simulink library "powerlib_modelsV2"  (Simulink 6.0)
settings: Solver=ode45  SolverMode=SingleTasking  StartTime=0.0  StopTime=10.0  RelTol=1e-3
values from neighbouring files (symbols this model uses):
  Ts = get(handles.edit1,'string')    [powergui.m]
undefined symbols (not defined in the file or in its folder): A, Ac, B, Bc, C, Cc, Cs, Current, damp, Dc, Dd, DiscIntNeverNeededParam, dref, dwo, exc, F, fb, gate, GH, GHd, GI, GId, GL, GLd, H, HT, hyd, ib, ib2, io, isfinite, j, K, Kd, Kg, L, Lad, Laq, lim, LIM, Ll, Llfd, Llkd, Llkq1, Llkq2, Llr, Lls, LowerFlux, N, N2, Nb, Nb2, nb_arm, p, Par_HarmoA_pu, Par_HarmoB_pu, Par_Timing_Harmo, Par_Timing_Variation, Par_Vps, Pb ... (+57)
libraries: powerlib_extras x14
(part 10 of 11)

== system powerlib_modelsV2/Switch Current Source/gto/Conduction Logic ==
  iak : Inport  Port=1  LatchInput=off
  Vak : Inport  Port=2  LatchInput=off
  g : Inport  Port=3  LatchInput=off
  "      " : Constant  Value=0
  ". " : Logic
  . 1 : Logic  Operator=OR
  Break Alg. Loop : Subsystem  mask{Nsw=length(Ron)}
      mask prompts: Nsw "number of switches"
  Data Type  Conversion{1..3,5..6} (5 alike) : DataTypeConversion  SaturateOnIntegerOverflow=on  RndMeth=Zero
  I>0 : Relay  OnSwitchValue=1000*eps  OffSwitchValue=0
  I>1.5 : Relay  OnSwitchValue=1.5  OffSwitchValue=0
  Test2 : Switch  Threshold=eps  InputSameDT=on
  Vf : Constant  Value=Vf
  b : RelationalOperator  Operator=>  InputSameDT=on
  n1 : Sum  SaturateOnIntegerOverflow=on  InputSameDT=on
  status : Outport  InitialOutput=0
  wires:
  Data Type  Conversion5/1 -> Test2/2, ". "/2
  Break Alg. Loop/1(Out1) -> Data Type  Conversion3/1, n1/2
  ". "/1 -> Break Alg. Loop/1(In1)
  Data Type  Conversion3/1 -> . 1/2
  Data Type  Conversion2/1 -> . 1/1
  I>1.5/1 -> Data Type  Conversion2/1
  Data Type  Conversion1/1 -> Test2/1
  . 1/1 -> Data Type  Conversion1/1
  n1/1 -> I>1.5/1
  iak/1 -> I>0/1
  I>0/1 -> n1/1
  Vf/1 -> b/2
  "      "/1 -> Test2/3
  Test2/1 -> status/1
  g/1 -> Data Type  Conversion5/1  "gate signal"
  Data Type  Conversion6/1 -> ". "/1
  b/1 -> Data Type  Conversion6/1
  Vak/1 -> b/1

== system powerlib_modelsV2/Switch Current Source/gto/Tail ==
  iak : Inport  Port=1  LatchInput=off
  switch : Inport  Port=2  LatchInput=off
  1 : Constant
  Integrator : Integrator  ExternalReset=falling  LimitOutput=on
  Look-Up  Table : Lookup  DialogController=Simulink.DDGSource  InputValues="[  0   Tf+eps Tf+Tt+2*eps  Tf+Tt+3*eps]"  OutputValues="[  1   0.1*(Tt>0) 0 0]"  SaturateOnIntegerOverflow=on
  Product : Product  SaturateOnIntegerOverflow=on  InputSameDT=on
  Switch : Switch  Threshold=eps  InputSameDT=on
  Iak : Outport  InitialOutput=0
  wires:
  iak/1 -> Product/1, Switch/1
  Look-Up  Table/1 -> Product/2
  switch/1 -> Switch/2, Integrator/2
  1/1 -> Integrator/1
  Integrator/1 -> Look-Up  Table/1
  Switch/1 -> Iak/1
  Product/1 -> Switch/3

== system powerlib_modelsV2/Switch Current Source/mosfet/Conduction Logic ==
  Ids_meas : Inport  Port=1  LatchInput=off
  Vds : Inport  Port=2  LatchInput=off
  G : Inport  Port=3  LatchInput=off
  "      1" : Constant
  . 1 : Logic  Operator=OR
  . 2 : Logic
  . 3 : Logic  Operator=NOT  Inputs=1
  Break Alg. Loop : Subsystem  mask{Nsw=length(Ron)}
      mask prompts: Nsw "number of switches"
  Data Type  Conversion{,1..2,4..5} (5 alike) : DataTypeConversion  SaturateOnIntegerOverflow=on  RndMeth=Zero
  Test2 : Switch  Threshold=eps  InputSameDT=on
  test_v : RelationalOperator  Operator=<  InputSameDT=on
  test_v1 : RelationalOperator  Operator=<  InputSameDT=on
  zero : Constant  Value=-eps
  zero1 : Constant  Value=-eps
  status : Outport  InitialOutput=0
  wires:
  Break Alg. Loop/1(Out1) -> Data Type  Conversion2/1
  "      1"/1 -> Test2/1
  Test2/1 -> status/1
  Data Type  Conversion/1 -> Test2/3
  test_v/1 -> Data Type  Conversion4/1
  Data Type  Conversion1/1 -> Test2/2, . 3/1
  Data Type  Conversion5/1 -> . 1/1
  test_v1/1 -> Data Type  Conversion5/1
  Data Type  Conversion4/1 -> . 2/1
  zero1/1 -> test_v1/2
  Ids_meas/1 -> test_v1/1
  zero/1 -> test_v/2
  . 2/1 -> Break Alg. Loop/1(In1)
  . 3/1 -> . 2/2
  . 1/1 -> Data Type  Conversion/1
  G/1 -> Data Type  Conversion1/1
  Vds/1 -> test_v/1
  Data Type  Conversion2/1 -> . 1/2

== system powerlib_modelsV2/Switch Current Source/thyristor/Conduction Logic ==
  "Iak " : Inport  Port=1  LatchInput=off
  Vak : Inport  Port=2  LatchInput=off
  "G " : Inport  Port=3  LatchInput=off
  0 1 : Constant  Value=0
  0 2 : Constant  Value=Vf
  0 3 : Constant  Value=0
  Break Alg. Loop : Subsystem  AncestorBlock=powerlib_models/Switch Current Source/thyristor/Conduction Logic/BAL-PB1  mask{Nsw=length(Lon), IC=IC}
      mask prompts: Nsw "number of switches"; IC "initial conditions"
  Data Type  Conversion{1..2,4,6} (4 alike) : DataTypeConversion  SaturateOnIntegerOverflow=on  RndMeth=Zero
  b5 : RelationalOperator  Operator=>  InputSameDT=on
  b6 : RelationalOperator  Operator=>  InputSameDT=on
  b7 : RelationalOperator  Operator===  InputSameDT=on
  or2 : Logic  Operator=OR
  or3 : Logic  Inputs=3
  Status : Outport  InitialOutput=0
  wires:
  Data Type  Conversion4/1 -> or3/3
  or3/1 -> or2/2
  or2/1 -> Break Alg. Loop/1(In1)
  b6/1 -> Data Type  Conversion2/1  "Voltage > Vf"
  b5/1 -> Data Type  Conversion1/1  "Current > 0"
  Vak/1 -> b6/1  "thyristor voltage"
  0 1/1 -> b5/2
  b7/1 -> Data Type  Conversion6/1  "Current = 0"
  0 3/1 -> b7/2
  0 2/1 -> b6/2
  "Iak "/1 -> b7/1, b5/1  "thyristor current"
  "G "/1 -> Data Type  Conversion4/1  "gate signal"
  Data Type  Conversion6/1 -> or3/2
  Data Type  Conversion1/1 -> or2/1
  Data Type  Conversion2/1 -> or3/1
  Break Alg. Loop/1(Out1) -> Status/1

== system powerlib_modelsV2/Continuous/Dynamic_Load/3-phase PLL1/2nd-Order Filter ==
  In : Inport  Port=1  LatchInput=off
  State-Space : StateSpace  A=Ac  B=Bc  C=Cc  D=Dc  X0=x0c
  Out : Outport  InitialOutput=0
  wires:
  State-Space/1 -> Out/1
  In/1 -> State-Space/1

== system powerlib_modelsV2/Continuous/Dynamic_Load/3-phase PLL1/Discrete PI Controller ==
  Error : Inport  Port=1  LatchInput=off
  Integrator : Integrator  InitialCondition=Init  LimitOutput=on  UpperSaturationLimit=UpperLimit  LowerSaturationLimit=LowerLimit
  Kp4 : Gain  Gain=Kp  SaturateOnIntegerOverflow=on
  Kp5 : Gain  Gain=Ki  SaturateOnIntegerOverflow=on
  Saturation2 : Saturate  UpperLimit=UpperLimit  LowerLimit=LowerLimit
  Sum6 : Sum  SaturateOnIntegerOverflow=on  InputSameDT=on
  Out : Outport  InitialOutput=0
  wires:
  Error/1 -> Kp4/1, Kp5/1
  Sum6/1 -> Saturation2/1
  Kp5/1 -> Integrator/1
  Kp4/1 -> Sum6/1
  Integrator/1 -> Sum6/2
  Saturation2/1 -> Out/1

== system powerlib_modelsV2/Continuous/Dynamic_Load/3-phase PLL1/Variable Frequency Mean value ==
  note: Mean Value (Variable frequency)
  note: Pierre Giroux, Gilbert Sybille
      | Power System Simulation Laboratory
      | IREQ, Hydro-Quebc
  Freq : Inport  Port=1  LatchInput=off
  In : Inport  Port=2  LatchInput=off
  Constant : Constant  Value=Vinit
  Integrator : Integrator
  Number of samples per cycle : Fcn  Expr=1/u[1]
  Product : Product  SaturateOnIntegerOverflow=on  InputSameDT=on
  Step : Step  Time=1/Finit  SampleTime=0
  Sum7 : Sum  Inputs=-+  SaturateOnIntegerOverflow=on  InputSameDT=on
  Switch : Switch  Threshold=0.5  InputSameDT=on
  To avoid division by zero : Saturate  Orientation=down  UpperLimit=1e6  LowerLimit=1e-6
  Variable Transport Delay : VariableTransportDelay  MaximumDelay=1/40  MaximumPoints=4096
  Mean : Outport
  wires:
  Number of samples per cycle/1 -> Variable Transport Delay/2  "Delay"
  Step/1 -> Switch/2
  To avoid division by zero/1 -> Number of samples per cycle/1  "Freq"
  Switch/1 -> Mean/1
  Constant/1 -> Switch/3
  Freq/1 -> To avoid division by zero/1, Product/2  "Freq"
  Integrator/1 -> Variable Transport Delay/1, Sum7/2
  Sum7/1 -> Product/1
  Variable Transport Delay/1 -> Sum7/1
  Product/1 -> Switch/1  "Mean value"
  In/1 -> Integrator/1  "In"

== system powerlib_modelsV2/Continuous/Dynamic_Load/3-phase PLL1/abc_to_dq1 ==
  note: This subsystem converts Vab and Vbc to Vd,Vq
  Vab_bc : Inport  Port=1  LatchInput=off
  sin_cos : Inport  Port=2  LatchInput=off
  Fcn2 : Fcn  Expr=(u[4]*(2*u[1]+u[2]) + (sqrt(3)*u[2]*u[3]))/3
  Fcn3 : Fcn  Expr=(u[3]*(2*u[1]+u[2]) + (-sqrt(3)*u[2]*u[4]))/3
  Mux1 : Mux  Inputs=[ 2 2 ]
  vd : Outport  InitialOutput=0
  vq : Outport  Port=2  InitialOutput=0
  wires:
  Vab_bc/1 -> Mux1/1
  Mux1/1 -> Fcn2/1, Fcn3/1
  sin_cos/1 -> Mux1/2
  Fcn2/1 -> vq/1
  Fcn3/1 -> vd/1

== system powerlib_modelsV2/Continuous/Dynamic_Load/Break  Alg. Loop/imag ==
  In1 : Inport  Port=1  LatchInput=off
  State Space : StateSpace  A=A  B=B  C=C  D=Dd  X0=X0
  Out1 : Outport  InitialOutput=0
  wires:
  In1/1 -> State Space/1
  State Space/1 -> Out1/1

== system powerlib_modelsV2/Continuous/Dynamic_Load/Break  Alg. Loop/real ==
  In1 : Inport  Port=1  LatchInput=off
  State Space : StateSpace  A=A  B=B  C=C  D=Dd  X0=X0
  Out1 : Outport  InitialOutput=0
  wires:
  In1/1 -> State Space/1
  State Space/1 -> Out1/1

== system powerlib_modelsV2/Continuous/Dynamic_Load/Positive Sequence  current/TF_P ==
  In1 : Inport  Port=1  LatchInput=off
  State-Space : StateSpace  A=Ac  B=Bc  C=Cc  D=Dc  X0=x0c
  Out1 : Outport
  wires:
  In1/1 -> State-Space/1
  State-Space/1 -> Out1/1

== system powerlib_modelsV2/Continuous/Dynamic_Load/Positive Sequence  current/TF_Q ==
  In1 : Inport  Port=1  LatchInput=off
  State-Space : StateSpace  A=Ac  B=Bc  C=Cc  D=Dc  X0=x0c
  Out1 : Outport
  wires:
  State-Space/1 -> Out1/1
  In1/1 -> State-Space/1

== system powerlib_modelsV2/Continuous/GTO-IGBT Bridge/Diode Logic/Blocking Diodes ==
  G : Inport  Port=1  LatchInput=off
  Bloque D214365 : Selector  Elements=Selec_Diode  InputPortWidth=nb_switch
  Logical Operator : Logic  Operator=NOT
  Memory : Memory  InheritSampleTime=on
  Pulse 1 step : Logic
  Block.D : Outport
  wires:
  Bloque D214365/1 -> Block.D/1
  Pulse 1 step/1 -> Bloque D214365/1  "Blockinkg"
  Memory/1 -> Logical Operator/1
  Logical Operator/1 -> Pulse 1 step/1
  G/1 -> Memory/1, Pulse 1 step/2

== system powerlib_modelsV2/Continuous/GTO-IGBT Bridge/Diode Logic/Trig.  Diodes (No Snubber Capacitance) ==
  G : Inport  Port=1  LatchInput=off
  Ipos : Inport  Port=2  LatchInput=off
  Enable : EnablePort  StatesWhenEnabling=reset
  Data Type  Conversion3 : DataTypeConversion  SaturateOnIntegerOverflow=on  RndMeth=Zero
  Logical Operator : Logic  Operator=NOT
  Memory : Memory  InheritSampleTime=on
  Pulse 1 step : Logic  Inputs=3
  Trig D214365 : Selector  Elements=Selec_Diode  InputPortWidth=nb_switch
  Trig D : Outport
  wires:
  Trig D214365/1 -> Trig D/1
  Pulse 1 step/1 -> Trig D214365/1
  Memory/1 -> Pulse 1 step/2
  Logical Operator/1 -> Pulse 1 step/1
  G/1 -> Memory/1, Logical Operator/1
  Ipos/1 -> Data Type  Conversion3/1
  Data Type  Conversion3/1 -> Pulse 1 step/3

== system powerlib_modelsV2/Continuous/MBPSS/Transfer function for detailed model (HF)/Transfer functions for detailed stabilizer ==
  In1 : Inport  Port=1  LatchInput=off
  Enable : EnablePort
  HF2 : TransferFcn  Numerator=[TH3 1]  Denominator=[TH4 1]
  HF3 : TransferFcn  Numerator=[TH5 1]  Denominator=[TH6 1]
  Out1 : Outport
  wires:
  In1/1 -> HF2/1
  HF3/1 -> Out1/1
  HF2/1 -> HF3/1

== system powerlib_modelsV2/Continuous/MBPSS/Transfer function for detailed model (HF)/Transfer functions for detailed stabilizer2 ==
  In1 : Inport  Port=1  LatchInput=off
  Enable : EnablePort
  HF5 : TransferFcn  Numerator=[TH9 1]  Denominator=[TH10 1]
  HF6 : TransferFcn  Numerator=[TH11 1]  Denominator=[TH12 1]
  Out1 : Outport
  wires:
  HF6/1 -> Out1/1
  In1/1 -> HF5/1
  HF5/1 -> HF6/1

== system powerlib_modelsV2/Continuous/MBPSS/Transfer function for detailed model (IF)/Transfer functions for detailed stabilizer ==
  In1 : Inport  Port=1  LatchInput=off
  Enable : EnablePort
  IF2 : TransferFcn  Numerator=[TI3 1]  Denominator=[TI4 1]
  IF3 : TransferFcn  Numerator=[TI5 1]  Denominator=[TI6 1]
  Out1 : Outport
  wires:
  IF3/1 -> Out1/1
  IF2/1 -> IF3/1
  In1/1 -> IF2/1

== system powerlib_modelsV2/Continuous/MBPSS/Transfer function for detailed model (IF)/Transfer functions for detailed stabilizer2 ==
  In1 : Inport  Port=1  LatchInput=off
  Enable : EnablePort
  IF5 : TransferFcn  Numerator=[TI9 1]  Denominator=[TI10 1]
  IF6 : TransferFcn  Numerator=[TI11 1]  Denominator=[TI12 1]
  Out1 : Outport
  wires:
  In1/1 -> IF5/1
  IF6/1 -> Out1/1
  IF5/1 -> IF6/1

== system powerlib_modelsV2/Continuous/MBPSS/Transfer function for detailed model (LF)/Transfer functions for detailed stabilizer ==
  In1 : Inport  Port=1  LatchInput=off
  Enable : EnablePort
  BF2 : TransferFcn  Numerator=[TL3 1]  Denominator=[TL4 1]
  BF3 : TransferFcn  Numerator=[TL5 1]  Denominator=[TL6 1]
  Out1 : Outport
  wires:
  BF2/1 -> BF3/1
  In1/1 -> BF2/1
  BF3/1 -> Out1/1

== system powerlib_modelsV2/Continuous/MBPSS/Transfer function for detailed model (LF)/Transfer functions for detailed stabilizer2 ==
  In1 : Inport  Port=1  LatchInput=off
  Enable : EnablePort
  BF5 : TransferFcn  Numerator=[TL9 1]  Denominator=[TL10 1]
  BF6 : TransferFcn  Numerator=[TL11 1]  Denominator=[TL12 1]
  Out1 : Outport
  wires:
  BF6/1 -> Out1/1
  In1/1 -> BF5/1
  BF5/1 -> BF6/1

== system powerlib_modelsV2/Continuous/PM_synchronous_machine/iq,id/id ==
  iq : Inport  Port=1  LatchInput=off
  we : Inport  Port=2  LatchInput=off
  vd : Inport  Port=3  LatchInput=off
  1/Ld : Gain  Gain=1/Ld  SaturateOnIntegerOverflow=on
  Lq/Ld : Gain  Gain=Lq/Ld  SaturateOnIntegerOverflow=on
  Product : Product  SaturateOnIntegerOverflow=on  InputSameDT=on
  R/Ld : Gain  Gain=R/Ld  SaturateOnIntegerOverflow=on
  Sum : Sum  Inputs=-++  SaturateOnIntegerOverflow=on  InputSameDT=on
  "id " : Integrator
  id : Outport  InitialOutput=0
  wires:
  1/Ld/1 -> Sum/2
  R/Ld/1 -> Sum/1
  Lq/Ld/1 -> Sum/3
  Sum/1 -> "id "/1
  Product/1 -> Lq/Ld/1
  "id "/1 -> R/Ld/1, id/1
  vd/1 -> 1/Ld/1
  we/1 -> Product/1
  iq/1 -> Product/2

== system powerlib_modelsV2/Continuous/PM_synchronous_machine/iq,id/iq ==
  vq : Inport  Port=1  LatchInput=off
  we : Inport  Port=2  LatchInput=off
  id : Inport  Port=3  LatchInput=off
  1/Lq : Gain  Gain=1/Lq  SaturateOnIntegerOverflow=on
  Ld/Lq : Gain  Gain=Ld/Lq  SaturateOnIntegerOverflow=on
  Product1 : Product  SaturateOnIntegerOverflow=on  InputSameDT=on
  R/Lq : Gain  Gain=R/Lq  SaturateOnIntegerOverflow=on
  Sum1 : Sum  Inputs=---+  SaturateOnIntegerOverflow=on  InputSameDT=on
  "iq " : Integrator
  lam/Lq : Gain  Gain=lam/Lq  SaturateOnIntegerOverflow=on
  iq : Outport  InitialOutput=0
  wires:
  R/Lq/1 -> Sum1/1
  Ld/Lq/1 -> Sum1/2
  lam/Lq/1 -> Sum1/3
  Sum1/1 -> "iq "/1
  Product1/1 -> Ld/Lq/1
  1/Lq/1 -> Sum1/4
  id/1 -> Product1/1
  vq/1 -> 1/Lq/1
  we/1 -> Product1/2, lam/Lq/1
  "iq "/1 -> R/Lq/1, iq/1

== system powerlib_modelsV2/Continuous/Three-Level Bridge/2-level GTO-IGBT Bridge  Logic (modified)/Diode Logic ==
  Vak : Inport  Port=1  LatchInput=off
  G : Inport  Port=2  LatchInput=off
  0 2 : Constant  Value=0
  1 : Logic
  Blocking Diodes : Subsystem
  Data Type  Conversion5 : DataTypeConversion  SaturateOnIntegerOverflow=on  RndMeth=Zero
  Logical Operator3 : Logic  Operator=NOT
  b6 : RelationalOperator  Operator=>  InputSameDT=on
  status : Outport  InitialOutput=0
  block : Outport  Port=2  InitialOutput=0
  wires:
  Data Type  Conversion5/1 -> 1/1
  b6/1 -> Data Type  Conversion5/1
  Vak/1 -> b6/1
  0 2/1 -> b6/2
  G/1 -> Blocking Diodes/1(G)
  Blocking Diodes/1(Block.D) -> Logical Operator3/1, block/1
  Logical Operator3/1 -> 1/2
  1/1 -> status/1

== system powerlib_modelsV2/Continuous/Three-Level Bridge/2-level GTO-IGBT Bridge  Logic (modified)/GTO Logic ==
  Vak : Inport  Port=1  LatchInput=off
  G : Inport  Port=2  LatchInput=off
  " " : RelationalOperator  Operator=>  InputSameDT=on
  "    " : Constant  Value=0
  ". " : Logic
  Data Type  Conversion1 : DataTypeConversion  SaturateOnIntegerOverflow=on  RndMeth=Zero
  Data Type  Conversion2 : DataTypeConversion  SaturateOnIntegerOverflow=on  RndMeth=Zero
  Data Type  Conversion3 : DataTypeConversion  SaturateOnIntegerOverflow=on  RndMeth=Zero
  Vpos : Constant  Value=0
  b : RelationalOperator  Operator=>  InputSameDT=on
  status : Outport  InitialOutput=0
  wires:
  Data Type  Conversion3/1 -> " "/2
  "    "/1 -> Data Type  Conversion3/1
  Data Type  Conversion2/1 -> ". "/2
  " "/1 -> Data Type  Conversion2/1
  Data Type  Conversion1/1 -> ". "/1
  b/1 -> Data Type  Conversion1/1
  G/1 -> " "/1
  Vpos/1 -> b/2
  Vak/1 -> b/1
  ". "/1 -> status/1

== system powerlib_modelsV2/Continuous/Three-Level Bridge/2-level GTO-IGBT Bridge  Logic (modified)/Vf  ==
  status_GTO : Inport  Port=1  LatchInput=off
  Switch : Switch  Threshold=0.5  SaturateOnIntegerOverflow=on  InputSameDT=on
  Vf device : Constant  Value=Vf*ones(nb_switch,1)
  Vf diode : Constant  Value=-Vfd*ones(nb_switch,1)
  Vf : Outport  InitialOutput=[0]
  wires:
  Vf device/1 -> Switch/1
  Vf diode/1 -> Switch/3
  Switch/1 -> Vf/1
  status_GTO/1 -> Switch/2

== system powerlib_modelsV2/Continuous/Three-Level Bridge/Sw3 (clamping diode) Logic/Note 3 ==
  G : Inport  Port=1  LatchInput=off
  Logical Operator : Logic  Operator=NOT
  Memory : Memory
  Mux : Mux  Inputs=[nb_arm nb_arm]
  Pulse 1 step : Logic
  Select_BlockD : Selector  Elements=BlockDElements  InputPortWidth=nb_arm*2
  Block.D : Outport
  wires:
  Select_BlockD/1 -> Block.D/1
  Mux/1 -> Select_BlockD/1
  Pulse 1 step/1 -> Mux/1, Mux/2  "Blocking"
  G/1 -> Memory/1, Pulse 1 step/2
  Logical Operator/1 -> Pulse 1 step/1
  Memory/1 -> Logical Operator/1

== system powerlib_modelsV2/Continuous/Three-Level Bridge/Sw3 (clamping diode) Logic/Note 4 ==
  pulses : Inport  Port=1  LatchInput=off
  D5_On : Inport  Port=2  LatchInput=off
  D6_On : Inport  Port=3  LatchInput=off
  Status_GTO : Inport  Port=4  LatchInput=off
  Demux : Demux  Outputs=[nb_arm nb_arm nb_arm nb_arm]
  Demux1 : Demux  Outputs=[nb_arm nb_arm]
  Logical Operator{,4,6,10} (4 alike) : Logic  Operator=NOT
  Logical Operator1 : Logic  Operator=NOR  Inputs=4
  Logical Operator{2..3,5,9} (4 alike) : Logic  Inputs=3
  Logical Operator7 : Logic  Operator=OR
  Logical Operator8 : Logic  Operator=OR
  Memory{,1..3} (4 alike) : Memory
  Mux1 : Mux  Inputs=2
  Select_StatGTO : Selector  Elements=Trig12Elements  InputPortWidth=nb_arm*2
  Trig12 : Outport
  wires:
  Logical Operator9/1 -> Logical Operator7/2
  Logical Operator2/1 -> Logical Operator8/2
  Memory3/1 -> Logical Operator9/2
  Demux1/2 -> Memory3/1, Logical Operator10/1
  Logical Operator10/1 -> Logical Operator9/3
  Demux1/1 -> Memory2/1, Logical Operator6/1
  Select_StatGTO/1 -> Demux1/1
  Logical Operator8/1 -> Mux1/2
  Logical Operator5/1 -> Logical Operator8/1
  Logical Operator7/1 -> Mux1/1
  Logical Operator3/1 -> Logical Operator7/1
  Memory2/1 -> Logical Operator2/2
  Logical Operator6/1 -> Logical Operator2/3
  Status_GTO/1 -> Select_StatGTO/1
  Logical Operator1/1 -> Logical Operator9/1, Logical Operator2/1, Logical Operator5/1, Logical Operator3/3
  Demux/4 -> Logical Operator1/4
  Demux/3 -> Logical Operator1/3
  Demux/2 -> Logical Operator1/2
  Demux/1 -> Logical Operator1/1
  Mux1/1 -> Trig12/1
  Logical Operator4/1 -> Logical Operator5/3
  Memory1/1 -> Logical Operator5/2
  D5_On/1 -> Memory1/1, Logical Operator4/1
  Logical Operator/1 -> Logical Operator3/2
  Memory/1 -> Logical Operator3/1
  D6_On/1 -> Memory/1, Logical Operator/1
  pulses/1 -> Demux/1

== system powerlib_modelsV2/Continuous/Three-Level Bridge/Sw3 (clamping diode) Logic/Vf Computation for Sw3 ==
  D5_On : Inport  Port=1  LatchInput=off
  Gain1 : Gain  Gain=-1  SaturateOnIntegerOverflow=on
  Gain2 : Gain  SaturateOnIntegerOverflow=on
  Switch : Switch  Threshold=0.5  SaturateOnIntegerOverflow=on  InputSameDT=on
  Vf device : Constant  Value=(Vf+Vfd)*ones(nb_arm,1)
  Vf : Outport
  wires:
  Switch/1 -> Vf/1
  Vf device/1 -> Gain1/1, Gain2/1
  Gain1/1 -> Switch/1
  Gain2/1 -> Switch/3
  D5_On/1 -> Switch/2

== system powerlib_modelsV2/Continuous/asynchronous_machine/abc2qd/Rotor reference frame ==
  In1 : Inport  Port=1  LatchInput=off
  Enable : EnablePort  StatesWhenEnabling=reset
  Mux2 : Mux  Inputs=2
  Mux3 : Mux  Inputs=2
  vdr : Fcn  Expr=-sqrt3_3 * u[2]
  vds : Fcn  Expr=one_third * (2*u[5]*u[3] + (u[5]-sqrt3*u[6]) * u[4])
  vqr : Fcn  Expr=one_third * (2*u[1] + u[2])
  vqs : Fcn  Expr=one_third * (2*u[6]*u[3] + (u[6]+sqrt3*u[5]) * u[4])
  vqr,vdr : Outport  OutputWhenDisabled=reset  InitialOutput=0
  vqs,vds : Outport  Port=2  OutputWhenDisabled=reset  InitialOutput=0
  wires:
  In1/1 -> vdr/1, vds/1, vqs/1, vqr/1
  Mux3/1 -> vqr,vdr/1  "Vqr,vdr"
  vqr/1 -> Mux3/1
  vdr/1 -> Mux3/2
  Mux2/1 -> vqs,vds/1  "Vqs,vds"
  vds/1 -> Mux2/2
  vqs/1 -> Mux2/1

== system powerlib_modelsV2/Continuous/asynchronous_machine/abc2qd/Stationary reference frame ==
  In1 : Inport  Port=1  LatchInput=off
  Enable : EnablePort  StatesWhenEnabling=reset
  Mux2 : Mux  Inputs=2
  Mux3 : Mux  Inputs=2
  vdr : Fcn  Expr=one_third * (-2*u[5]*u[1] + (-u[5]-sqrt3*u[6]) * u[2])
  vds : Fcn  Expr=-sqrt3_3*u[4]
  vqr : Fcn  Expr=one_third * (2*u[6]*u[1] + (u[6]-sqrt3*u[5]) * u[2])
  vqs : Fcn  Expr=one_third * (2*u[3] + u[4])
  vqr,vdr : Outport  OutputWhenDisabled=reset  InitialOutput=0
  vqs,vds : Outport  Port=2  OutputWhenDisabled=reset  InitialOutput=0
  wires:
  Mux3/1 -> vqr,vdr/1  "Vqr,vdr"
  In1/1 -> vdr/1, vqs/1, vds/1, vqr/1
  vdr/1 -> Mux3/2
  vqr/1 -> Mux3/1
  Mux2/1 -> vqs,vds/1  "Vqs,vds"
  vqs/1 -> Mux2/1
  vds/1 -> Mux2/2

== system powerlib_modelsV2/Continuous/asynchronous_machine/abc2qd/Synchronous reference frame ==
  In1 : Inport  Port=1  LatchInput=off
  Enable : EnablePort  StatesWhenEnabling=reset
  Mux2 : Mux  Inputs=2
  Mux3 : Mux  Inputs=2
  vdr : Fcn  Expr=(2*u[5]*u[1] + (u[5]-sqrt3*u[6]) * u[2]) / 3
  vds : Fcn  Expr=(2*u[7]*u[3] + (u[7]-sqrt3*u[8]) * u[4]) / 3
  vqr : Fcn  Expr=(2*u[6]*u[1] + (u[6]+sqrt3*u[5]) * u[2]) / 3
  vqs : Fcn  Expr=(2*u[8]*u[3] + (u[8]+sqrt3*u[7]) * u[4]) / 3
  vqr,vdr : Outport  OutputWhenDisabled=reset  InitialOutput=0
  vqs,vds : Outport  Port=2  OutputWhenDisabled=reset  InitialOutput=0
  wires:
  Mux3/1 -> vqr,vdr/1  "Vqr,vdr"
  In1/1 -> vdr/1, vqs/1, vds/1, vqr/1
  vdr/1 -> Mux3/2
  vqr/1 -> Mux3/1
  Mux2/1 -> vqs,vds/1  "Vqs,vds"
  vds/1 -> Mux2/2
  vqs/1 -> Mux2/1

== system powerlib_modelsV2/Continuous/asynchronous_machine/abc2qd/transit ==
  vu : Inport  Port=1  LatchInput=off
  Constant6 : Constant  Value=[0;0]
  Mux1 : Mux  Inputs=2
  Selector : Selector  Elements=elements1  InputPortWidth=selWidth
  vr,vs : Outport
  wires:
  Selector/1 -> vr,vs/1
  vu/1 -> Mux1/2
  Mux1/1 -> Selector/1
  Constant6/1 -> Mux1/1

== system powerlib_modelsV2/Continuous/asynchronous_machine/dq2abc/Rotor reference frame ==
  In1 : Inport  Port=1  LatchInput=off
  Enable : EnablePort  StatesWhenEnabling=reset
  Mux1 : Mux  Inputs=2
  Mux2 : Mux  Inputs=2
  ira : Fcn  Expr=u[1]
  irb : Fcn  Expr=-(u[1] + sqrt3*u[2]) / 2
  isa : Fcn  Expr=u[6]*u[3]+u[5]*u[4]
  isb : Fcn  Expr=((-u[6]+sqrt3*u[5])*u[3] + (-sqrt3*u[6]-u[5])*u[4]) / 2
  ira,irb : Outport  OutputWhenDisabled=reset  InitialOutput=0
  isa,isb : Outport  Port=2  OutputWhenDisabled=reset  InitialOutput=0
  wires:
  Mux2/1 -> isa,isb/1  "isa,isb"
  Mux1/1 -> ira,irb/1  "ira,irb"
  In1/1 -> isb/1, isa/1, irb/1, ira/1
  isb/1 -> Mux2/2
  isa/1 -> Mux2/1
  irb/1 -> Mux1/2
  ira/1 -> Mux1/1

== system powerlib_modelsV2/Continuous/asynchronous_machine/dq2abc/Stationary reference frame ==
  In1 : Inport  Port=1  LatchInput=off
  Enable : EnablePort  StatesWhenEnabling=reset
  Mux1 : Mux  Inputs=2
  Mux2 : Mux  Inputs=2
  ira : Fcn  Expr=u[6]*u[1] - u[5]*u[2]
  irb : Fcn  Expr=((-u[6]-sqrt3*u[5])*u[1] + (u[5]-sqrt3*u[6])*u[2]) / 2
  isa : Fcn  Expr=u[3]
  isb : Fcn  Expr=-(u[3] + sqrt3*u[4]) / 2
  ira,irb : Outport  OutputWhenDisabled=reset  InitialOutput=0
  isa,isb : Outport  Port=2  OutputWhenDisabled=reset  InitialOutput=0
  wires:
  Mux2/1 -> isa,isb/1  "isa,isb"
  Mux1/1 -> ira,irb/1  "ira,irb"
  In1/1 -> isb/1, isa/1, irb/1, ira/1
  isb/1 -> Mux2/2
  isa/1 -> Mux2/1
  irb/1 -> Mux1/2
  ira/1 -> Mux1/1

== system powerlib_modelsV2/Continuous/asynchronous_machine/dq2abc/Synchronous reference frame ==
  In1 : Inport  Port=1  LatchInput=off
  Enable : EnablePort  StatesWhenEnabling=reset
  Mux1 : Mux  Inputs=2
  Mux2 : Mux  Inputs=2
  ira : Fcn  Expr=u[6]*u[1] + u[5]*u[2]
  irb : Fcn  Expr=((-u[6]+sqrt3*u[5])*u[1] + (-sqrt3*u[6]-u[5])*u[2]) / 2
  isa : Fcn  Expr=u[8]*u[3] + u[7]*u[4]
  isb : Fcn  Expr=((-u[8]+sqrt3*u[7])*u[3] + (-sqrt3*u[8]-u[7])*u[4]) / 2
  ira,irb : Outport  OutputWhenDisabled=reset  InitialOutput=0
  isa,isb : Outport  Port=2  OutputWhenDisabled=reset  InitialOutput=0
  wires:
  Mux2/1 -> isa,isb/1  "isa,isb"
  Mux1/1 -> ira,irb/1  "ira,irb"
  In1/1 -> isb/1, isa/1, irb/1, ira/1
  isb/1 -> Mux2/2
  isa/1 -> Mux2/1
  irb/1 -> Mux1/2
  ira/1 -> Mux1/1

== system powerlib_modelsV2/Continuous/asynchronous_machine/sin,cos/sin(beta),cos(beta),sin(th),cos(th) ==
  thr,wr : Inport  Port=1  LatchInput=off
  Enable : EnablePort  StatesWhenEnabling=reset
  Clock : Clock
      settings: Decimation=10
  Demux2 : Demux  Outputs=2
  Mux1 : Mux
  Sum : Sum  Inputs=-+|  SaturateOnIntegerOverflow=on  InputSameDT=on
  Sum1 : Sum  Inputs=|-+  SaturateOnIntegerOverflow=on  InputSameDT=on
  Trigonometric Function : Trigonometry
  Trigonometric Function1 : Trigonometry
  Trigonometric Function2 : Trigonometry  Operator=cos
  Trigonometric Function3 : Trigonometry  Operator=cos
  we : Constant
  web_psb : Gain  Gain=web_psb  SaturateOnIntegerOverflow=on
  "sin(beta),cos(beta), sin(th),cos(th)" : Outport  OutputWhenDisabled=reset  InitialOutput=0
  we-wr : Outport  Port=2  OutputWhenDisabled=reset  InitialOutput=0
  wires:
  thr,wr/1 -> Demux2/1
  Demux2/2 -> Sum/1  "wr"
  Trigonometric Function1/1 -> Mux1/1
  Trigonometric Function2/1 -> Mux1/2
  Trigonometric Function/1 -> Mux1/3
  Trigonometric Function3/1 -> Mux1/4
  Mux1/1 -> "sin(beta),cos(beta), sin(th),cos(th)"/1
  Sum1/1 -> Trigonometric Function1/1, Trigonometric Function2/1  "beta"
  Demux2/1 -> Sum1/1  "thr"
  web_psb/1 -> Sum1/2, Trigonometric Function/1, Trigonometric Function3/1  "th"
  Clock/1 -> web_psb/1
  Sum/1 -> we-wr/1  "we-wr"
  we/1 -> Sum/2

== system powerlib_modelsV2/Continuous/asynchronous_machine/sin,cos/sin(thr),cos(thr) ==
  thr : Inport  Port=1  LatchInput=off
  Enable : EnablePort  StatesWhenEnabling=reset
  Constant : Constant  Value=[0; 0]
  Mux2 : Mux  Inputs=3
  Trigonometric Function : Trigonometry
  Trigonometric Function1 : Trigonometry  Operator=cos
  sin(thr),cos(thr) : Outport  OutputWhenDisabled=reset  InitialOutput=0
  wires:
  Trigonometric Function/1 -> Mux2/1
  Trigonometric Function1/1 -> Mux2/2
  Constant/1 -> Mux2/3
  thr/1 -> Trigonometric Function/1, Trigonometric Function1/1
  Mux2/1 -> sin(thr),cos(thr)/1

== system powerlib_modelsV2/Continuous/simplified_sync_mach/Vt/LL2LN ==
  In1 : Inport  Port=1  LatchInput=off
  Enable : EnablePort
  Fcn : Fcn  Expr=(2*u(1)+u(2))/3
  Fcn1 : Fcn  Expr=(u(2)-u(1))/3
  Mux1 : Mux  Inputs=3
  Sum1 : Sum  Orientation=down  Inputs=--  SaturateOnIntegerOverflow=on  InputSameDT=on
  Out1 : Outport  OutputWhenDisabled=reset  InitialOutput=[0 0 0]
  wires:
  Sum1/1 -> Mux1/3
  Fcn1/1 -> Sum1/1, Mux1/2
  Fcn/1 -> Sum1/2, Mux1/1
  Mux1/1 -> Out1/1
  In1/1 -> Fcn/1, Fcn1/1

== system powerlib_modelsV2/Continuous/synchronous_machine/Delta angle/Cartesian to Polar ==
  x : Inport  Port=1  LatchInput=off
  y : Inport  Port=2  LatchInput=off
  Mux : Mux  Inputs=2
  x->r : Fcn  Expr=hypot(u[1],u[2])
  x->theta : Fcn  Expr=atan2(u[2],u[1])
  r : Outport  InitialOutput=0
  theta : Outport  Port=2  InitialOutput=0
  wires:
  Mux/1 -> x->theta/1, x->r/1
  x->r/1 -> r/1
  x/1 -> Mux/1
  y/1 -> Mux/2
  x->theta/1 -> theta/1

== system powerlib_modelsV2/Continuous/synchronous_machine/Delta angle/Radians to Degrees ==
  Radians in : Inport  Port=1  LatchInput=off
  Gain : Gain  Gain=180/pi  SaturateOnIntegerOverflow=on
  Degrees out : Outport  InitialOutput=0
  wires:
  Gain/1 -> Degrees out/1
  Radians in/1 -> Gain/1

== system powerlib_modelsV2/Continuous/synchronous_machine/currents and mutual fluxes/Saturation ==
  phimq_in : Inport  Port=1  LatchInput=off
  phimd_in : Inport  Port=2  LatchInput=off
  Data Type  Conversion{,1..4} (5 alike) : DataTypeConversion  SaturateOnIntegerOverflow=on  RndMeth=Zero
  Gain : Gain  Gain=2  SaturateOnIntegerOverflow=on
  Gain1 : Gain  Gain=3  SaturateOnIntegerOverflow=on
  Logical Operator : Logic  Operator=NOT  Inputs=1
  Logical Operator1 : Logic  Operator=NOT  Inputs=1
  Logical Operator2 : Logic
  Logical Operator3 : Logic  Orientation=down
  Multiport Switch : MultiPortSwitch  Inputs=3  InputSameDT=on
  Sum : Sum  Inputs=+++  SaturateOnIntegerOverflow=on  InputSameDT=on
  Switch : Switch  Threshold=0.5  InputSameDT=on
  Vs4 : Constant  Value=phis==1e6
  Vs5 : Constant  Value=isinf(Llkq2)
  d axis saturation : Subsystem  TreatAsAtomicUnit=on
  dq axis saturation : Subsystem  TreatAsAtomicUnit=on
  phimq_out : Outport
  phimd_out : Outport  Port=2
  wires:
  Data Type  Conversion4/1 -> Gain1/1
  Data Type  Conversion3/1 -> Logical Operator3/1, Logical Operator1/1
  Vs5/1 -> Data Type  Conversion3/1
  Data Type  Conversion1/1 -> Gain/1, d axis saturation/Enable
  Logical Operator3/1 -> Data Type  Conversion1/1
  Data Type  Conversion/1 -> Switch/2, Sum/1, dq axis saturation/Enable
  Logical Operator2/1 -> Data Type  Conversion/1
  Switch/1 -> phimq_out/1
  Multiport Switch/1 -> phimd_out/1
  Logical Operator/1 -> Logical Operator3/2, Logical Operator2/1
  Logical Operator1/1 -> Logical Operator2/2
  Gain1/1 -> Sum/3
  d axis saturation/1(phimd sat.) -> Multiport Switch/3  "phimds"
  dq axis saturation/2(phimd sat.) -> Multiport Switch/2
  Sum/1 -> Multiport Switch/1
  Gain/1 -> Sum/2
  phimq_in/1 -> Switch/3, dq axis saturation/2(phimq)
  dq axis saturation/1(phimq sat.) -> Switch/1
  phimd_in/1 -> Multiport Switch/4, d axis saturation/1(phimd), dq axis saturation/1(phimd)
  Data Type  Conversion2/1 -> Logical Operator/1
  Vs4/1 -> Data Type  Conversion2/1, Data Type  Conversion4/1

== system powerlib_modelsV2/Continuous/synchronous_machine/phikq2/Enabled integrator ==
  In1 : Inport  Port=1  LatchInput=off
  Enable : EnablePort
  int : Integrator  InitialCondition=phikq2o
  Out1 : Outport  InitialOutput=phikq2o
  wires:
  int/1 -> Out1/1
  In1/1 -> int/1

== system powerlib_modelsV2/Discrete/Dynamic_Load/Discrete 3-phase PLL/abc_to_dq1 ==
  note: This subsystem converts Vab and Vbc to Vd,Vq
  Vab_bc : Inport  Port=1  PortDimensions=2  LatchInput=off
  sin_cos : Inport  Port=2  PortDimensions=2  LatchInput=off
  Fcn2 : Fcn  Expr=(u[4]*(2*u[1]+u[2]) + (sqrt(3)*u[2]*u[3]))/3
  Fcn3 : Fcn  Expr=(u[3]*(2*u[1]+u[2]) + (-sqrt(3)*u[2]*u[4]))/3
  Mux1 : Mux  Inputs=[ 2 2 ]
  vd : Outport  InitialOutput=0
  vq : Outport  Port=2  InitialOutput=0
  wires:
  Vab_bc/1 -> Mux1/1
  Mux1/1 -> Fcn2/1, Fcn3/1
  sin_cos/1 -> Mux1/2
  Fcn2/1 -> vq/1
  Fcn3/1 -> vd/1

== system powerlib_modelsV2/Discrete/GTO-IGBT Bridge/Diode Logic/Blocking Diodes ==
  G : Inport  Port=1  LatchInput=off
  Bloque D214365 : Selector  Elements=Selec_Diode  InputPortWidth=nb_switch
  Logical Operator : Logic  Operator=NOT
  Pulse 1 step : Logic
  Unit Delay : UnitDelay  SampleTime=Ts
  Block.D : Outport
  wires:
  Bloque D214365/1 -> Block.D/1
  Pulse 1 step/1 -> Bloque D214365/1  "Blockinkg"
  Unit Delay/1 -> Logical Operator/1
  Logical Operator/1 -> Pulse 1 step/1
  G/1 -> Unit Delay/1, Pulse 1 step/2

== system powerlib_modelsV2/Discrete/GTO-IGBT Bridge/Diode Logic/Trig.  Diodes (No Snubber Capacitance) ==
  G : Inport  Port=1  LatchInput=off
  Ipos : Inport  Port=2  LatchInput=off
  Enable : EnablePort  StatesWhenEnabling=reset
  Data Type  Conversion5 : DataTypeConversion  SaturateOnIntegerOverflow=on  RndMeth=Zero
  Logical Operator : Logic  Operator=NOT
  Pulse 1 step : Logic  Inputs=3
  Trig D214365 : Selector  Elements=Selec_Diode  InputPortWidth=nb_switch
  Unit Delay1 : UnitDelay  SampleTime=Ts
  Trig D : Outport
  wires:
  Trig D214365/1 -> Trig D/1
  Pulse 1 step/1 -> Trig D214365/1
  Unit Delay1/1 -> Pulse 1 step/2
  Logical Operator/1 -> Pulse 1 step/1
  G/1 -> Unit Delay1/1, Logical Operator/1
  Ipos/1 -> Data Type  Conversion5/1
  Data Type  Conversion5/1 -> Pulse 1 step/3

== system powerlib_modelsV2/Discrete/HTG/servo-motor/servo-motor ==
  In : Inport  Port=1  LatchInput=off
  1st order Lowpass : Subsystem  AncestorBlock=|  mask(Discrete 1st-Order Filter){FilterType=Lowpass, Tc=ta, Ts=Ts, Initialize=off, Vac_Init=[0.8 -25 60], Vdc_Init=-0.4, PlotResponse=off, param1=[1 500 0.1]}
      | powerlib_extras/Discrete 
      | Control Blocks/Discrete
      | 1st-Order
      | Discrete Filter
      mask prompts: FilterType "Filter Type:"; Tc "Time constant (s):"; Ts "Sample time:"; Initialize "Initialize filter states"; Vac_Init "AC initial input: [ Mag  Phase(degrees)  Freq(Hz) ]"; Vdc_Init "DC Initial input:"; PlotResponse "Plot filter response"; param1 "Frequency range(Hz) : [Start  End  Inc.]"
      mask init: same as powerlib_modelsV2/Discrete/PSS/Sensor 
      mask StyleString: popup(Lowpass|Highpass),edit,edit,checkbox,edit,edit,checkbox,edit
      mask CallbackString: |||p4=get_param(gcb,'Initialize');if strcmp(p4,'on');visible={'on','on','on','on','on','on','on',get_param(gcb,'PlotResponse')};else;visible={'on','on','on','on','off','off','on',get_param(gcb,'PlotResponse')};end;set_param(gcb,'MaskVisibilities',visible)|||p7=get_param(gcb,'PlotResponse');if strcmp(p7,'on');visible={'on','on','on','on',get_param(gcb,'Initialize'),get_param(gcb,'Initialize'),'on','on'};else;visible={'on','on','on','on',get_param(gcb,'Initialize'),get_param(gcb,'Initialize'),'on','off'};end;set_param(gcb,'MaskVisibilities',visible)|
      mask Display: plot(X,Y);
  Gain : Gain  Gain=ka  SaturateOnIntegerOverflow=on
  Out : Outport
  wires:
  Gain/1 -> 1st order Lowpass/1(In)
  In/1 -> Gain/1
  1st order Lowpass/1(Out) -> Out/1

== system powerlib_modelsV2/Discrete/MBPSS/Transfer function for detailed model (HF)/Transfer functions for detailed stabilizer ==
  In1 : Inport  Port=1  LatchInput=off
  Enable : EnablePort
  Discrete Lead-Lag1 : Subsystem  mask(Discrete Lead-Lag Compensator){values=[TH3 TH4], Ts=Ts}
      mask prompts: values "Time constants (s): [ T1 T2 ]"; Ts "Sample time (s):"
      mask help:
      | This block implements a discrete lead-lag compensator:
      |
      |            T1.s + 1
      | H(s)=  -------
      |            T2.s + 1
      mask init:
      | numc=[values(1) 1];
      | denc=[values(2) 1];
      | [Ac,Bc,Cc,Dc]=tf2ss(numc,denc);
      | %
      | %  Conversion to discrete transfer function
      | nstates = size(Ac,1);
      | invexp = inv(eye(nstates) - (Ts/2)*Ac);
      | Ad = invexp*(eye(nstates) + (Ts/2)*Ac);
      | Bd = invexp*Bc;
      | Cd = Cc*invexp*Ts;
      | Dd = Cc*invexp*Bc*(Ts/2) + Dc;
      | %
      | if values(1)==0 & values(2)==0, Dd=1; end
      mask Display: disp('TH3.s+1\n---\nTH4.s+1')
  Discrete Lead-Lag2 : Subsystem  mask(Discrete Lead-Lag Compensator){values=[TH5 TH6], Ts=Ts}
      mask prompts: values "Time constants (s): [ T1 T2 ]"; Ts "Sample time (s):"
      mask help:
      | This block implements a discrete lead-lag compensator:
      |
      |            T1.s + 1
      | H(s)=  -------
      |            T2.s + 1
      mask init: same as powerlib_modelsV2/Discrete/MBPSS/Transfer function for detailed model (HF)/Transfer functions for detailed stabilizer/Discrete Lead-Lag1
      mask Display: disp('TH5.s+1\n---\nTH6.s+1')
  Out1 : Outport
  wires:
  Discrete Lead-Lag1/1(Out1) -> Discrete Lead-Lag2/1(In1)
  Discrete Lead-Lag2/1(Out1) -> Out1/1
  In1/1 -> Discrete Lead-Lag1/1(In1)

== system powerlib_modelsV2/Discrete/MBPSS/Transfer function for detailed model (HF)/Transfer functions for detailed stabilizer1 ==
  In1 : Inport  Port=1  LatchInput=off
  Enable : EnablePort
  Discrete Lead-Lag1 : Subsystem  mask(Discrete Lead-Lag Compensator){values=[TH9 TH10], Ts=Ts}
      mask prompts: values "Time constants (s): [ T1 T2 ]"; Ts "Sample time (s):"
      mask help:
      | This block implements a discrete lead-lag compensator:
      |
      |            T1.s + 1
      | H(s)=  -------
      |            T2.s + 1
      mask init: same as powerlib_modelsV2/Discrete/MBPSS/Transfer function for detailed model (HF)/Transfer functions for detailed stabilizer/Discrete Lead-Lag1
      mask Display: disp('TH9.s+1\n---\nTH10.s+1')
  Discrete Lead-Lag2 : Subsystem  mask(Discrete Lead-Lag Compensator){values=[TH11 TH12], Ts=Ts}
      mask prompts: values "Time constants (s): [ T1 T2 ]"; Ts "Sample time (s):"
      mask help:
      | This block implements a discrete lead-lag compensator:
      |
      |            T1.s + 1
      | H(s)=  -------
      |            T2.s + 1
      mask init: same as powerlib_modelsV2/Discrete/MBPSS/Transfer function for detailed model (HF)/Transfer functions for detailed stabilizer/Discrete Lead-Lag1
      mask Display: disp('TH11.s+1\n---\nTH12.s+1')
  Out1 : Outport
  wires:
  In1/1 -> Discrete Lead-Lag1/1(In1)
  Discrete Lead-Lag2/1(Out1) -> Out1/1
  Discrete Lead-Lag1/1(Out1) -> Discrete Lead-Lag2/1(In1)

== system powerlib_modelsV2/Discrete/MBPSS/Transfer function for detailed model (IF)/Transfer functions for detailed stabilizer ==
  In1 : Inport  Port=1  LatchInput=off
  Enable : EnablePort
  Discrete Lead-Lag1 : Subsystem  mask(Discrete Lead-Lag Compensator){values=[TI3 TI4], Ts=Ts}
      mask prompts: values "Time constants (s): [ T1 T2 ]"; Ts "Sample time (s):"
      mask help:
      | This block implements a discrete lead-lag compensator:
      |
      |            T1.s + 1
      | H(s)=  -------
      |            T2.s + 1
      mask init: same as powerlib_modelsV2/Discrete/MBPSS/Transfer function for detailed model (HF)/Transfer functions for detailed stabilizer/Discrete Lead-Lag1
      mask Display: disp('TI3.s+1\n---\nTI4.s+1')
  Discrete Lead-Lag2 : Subsystem  mask(Discrete Lead-Lag Compensator){values=[TI5 TI6], Ts=Ts}
      mask prompts: values "Time constants (s): [ T1 T2 ]"; Ts "Sample time (s):"
      mask help:
      | This block implements a discrete lead-lag compensator:
      |
      |            T1.s + 1
      | H(s)=  -------
      |            T2.s + 1
      mask init: same as powerlib_modelsV2/Discrete/MBPSS/Transfer function for detailed model (HF)/Transfer functions for detailed stabilizer/Discrete Lead-Lag1
      mask Display: disp('TI5.s+1\n---\nTI6.s+1')
  Out1 : Outport
  wires:
  In1/1 -> Discrete Lead-Lag1/1(In1)
  Discrete Lead-Lag2/1(Out1) -> Out1/1
  Discrete Lead-Lag1/1(Out1) -> Discrete Lead-Lag2/1(In1)

== system powerlib_modelsV2/Discrete/MBPSS/Transfer function for detailed model (IF)/Transfer functions for detailed stabilizer1 ==
  In1 : Inport  Port=1  LatchInput=off
  Enable : EnablePort
  Discrete Lead-Lag1 : Subsystem  mask(Discrete Lead-Lag Compensator){values=[TI9 TI10], Ts=Ts}
      mask prompts: values "Time constants (s): [ T1 T2 ]"; Ts "Sample time (s):"
      mask help:
      | This block implements a discrete lead-lag compensator:
      |
      |            T1.s + 1
      | H(s)=  -------
      |            T2.s + 1
      mask init: same as powerlib_modelsV2/Discrete/MBPSS/Transfer function for detailed model (HF)/Transfer functions for detailed stabilizer/Discrete Lead-Lag1
      mask Display: disp('TI9.s+1\n---\nTI10.s+1')
  Discrete Lead-Lag2 : Subsystem  mask(Discrete Lead-Lag Compensator){values=[TI11 TI12], Ts=Ts}
      mask prompts: values "Time constants (s): [ T1 T2 ]"; Ts "Sample time (s):"
      mask help:
      | This block implements a discrete lead-lag compensator:
      |
      |            T1.s + 1
      | H(s)=  -------
      |            T2.s + 1
      mask init: same as powerlib_modelsV2/Discrete/MBPSS/Transfer function for detailed model (HF)/Transfer functions for detailed stabilizer/Discrete Lead-Lag1
      mask Display: disp('TI11.s+1\n---\nTI12.s+1')
  Out1 : Outport
  wires:
  Discrete Lead-Lag1/1(Out1) -> Discrete Lead-Lag2/1(In1)
  Discrete Lead-Lag2/1(Out1) -> Out1/1
  In1/1 -> Discrete Lead-Lag1/1(In1)

== system powerlib_modelsV2/Discrete/MBPSS/Transfer function for detailed model (LF)/Transfer functions for detailed stabilizer ==
  In1 : Inport  Port=1  LatchInput=off
  Enable : EnablePort
  Discrete Lead-Lag1 : Subsystem  mask(Discrete Lead-Lag Compensator){values=[TL3 TL4], Ts=Ts}
      mask prompts: values "Time constants (s): [ T1 T2 ]"; Ts "Sample time (s):"
      mask help:
      | This block implements a discrete lead-lag compensator:
      |
      |            T1.s + 1
      | H(s)=  -------
      |            T2.s + 1
      mask init: same as powerlib_modelsV2/Discrete/MBPSS/Transfer function for detailed model (HF)/Transfer functions for detailed stabilizer/Discrete Lead-Lag1
      mask Display: disp('TL3.s+1\n---\nTL4.s+1')
  Discrete Lead-Lag2 : Subsystem  mask(Discrete Lead-Lag Compensator){values=[TL5 TL6], Ts=Ts}
      mask prompts: values "Time constants (s): [ T1 T2 ]"; Ts "Sample time (s):"
      mask help:
      | This block implements a discrete lead-lag compensator:
      |
      |            T1.s + 1
      | H(s)=  -------
      |            T2.s + 1
      mask init: same as powerlib_modelsV2/Discrete/MBPSS/Transfer function for detailed model (HF)/Transfer functions for detailed stabilizer/Discrete Lead-Lag1
      mask Display: disp('TL5.s+1\n---\nTL6.s+1')
  Out1 : Outport
  wires:
  Discrete Lead-Lag1/1(Out1) -> Discrete Lead-Lag2/1(In1)
  Discrete Lead-Lag2/1(Out1) -> Out1/1
  In1/1 -> Discrete Lead-Lag1/1(In1)

== system powerlib_modelsV2/Discrete/MBPSS/Transfer function for detailed model (LF)/Transfer functions for detailed stabilizer1 ==
  In1 : Inport  Port=1  LatchInput=off
  Enable : EnablePort
  Discrete Lead-Lag1 : Subsystem  mask(Discrete Lead-Lag Compensator){values=[TL9 TL10], Ts=Ts}
      mask prompts: values "Time constants (s): [ T1 T2 ]"; Ts "Sample time (s):"
      mask help:
      | This block implements a discrete lead-lag compensator:
      |
      |            T1.s + 1
      | H(s)=  -------
      |            T2.s + 1
      mask init: same as powerlib_modelsV2/Discrete/MBPSS/Transfer function for detailed model (HF)/Transfer functions for detailed stabilizer/Discrete Lead-Lag1
      mask Display: disp('TL9.s+1\n---\nTL10.s+1')
  Discrete Lead-Lag2 : Subsystem  mask(Discrete Lead-Lag Compensator){values=[TL11 TL12], Ts=Ts}
      mask prompts: values "Time constants (s): [ T1 T2 ]"; Ts "Sample time (s):"
      mask help:
      | This block implements a discrete lead-lag compensator:
      |
      |            T1.s + 1
      | H(s)=  -------
      |            T2.s + 1
      mask init: same as powerlib_modelsV2/Discrete/MBPSS/Transfer function for detailed model (HF)/Transfer functions for detailed stabilizer/Discrete Lead-Lag1
      mask Display: disp('TL11.s+1\n---\nTL12.s+1')
  Out1 : Outport
  wires:
  In1/1 -> Discrete Lead-Lag1/1(In1)
  Discrete Lead-Lag2/1(Out1) -> Out1/1
  Discrete Lead-Lag1/1(Out1) -> Discrete Lead-Lag2/1(In1)

== system powerlib_modelsV2/Discrete/PM_synchronous_machine/iq,id/id ==
  iq : Inport  Port=1  LatchInput=off
  we : Inport  Port=2  LatchInput=off
  vd : Inport  Port=3  LatchInput=off
  1/Ld : Gain  Gain=1/Ld  SaturateOnIntegerOverflow=on
  Discrete-Time Integrator : DiscreteIntegrator  SampleTime=Ts  SaturateOnIntegerOverflow=on  ICPrevOutput=DiscIntNeverNeededParam  ICPrevScaledInput=DiscIntNeverNeededParam
  Lq/Ld : Gain  Gain=Lq/Ld  SaturateOnIntegerOverflow=on
  Product : Product  SaturateOnIntegerOverflow=on  InputSameDT=on
  R/Ld : Gain  Gain=R/Ld  SaturateOnIntegerOverflow=on
  Sum : Sum  Inputs=-++  SaturateOnIntegerOverflow=on  InputSameDT=on
  id : Outport  InitialOutput=0
  wires:
  iq/1 -> Product/2
  we/1 -> Product/1
  vd/1 -> 1/Ld/1
  Discrete-Time Integrator/1 -> id/1, R/Ld/1
  Product/1 -> Lq/Ld/1
  Sum/1 -> Discrete-Time Integrator/1
  Lq/Ld/1 -> Sum/3
  R/Ld/1 -> Sum/1
  1/Ld/1 -> Sum/2

== system powerlib_modelsV2/Discrete/PM_synchronous_machine/iq,id/iq ==
  vq : Inport  Port=1  LatchInput=off
  we : Inport  Port=2  LatchInput=off
  id : Inport  Port=3  LatchInput=off
  1/Lq : Gain  Gain=1/Lq  SaturateOnIntegerOverflow=on
  Discrete-Time Integrator : DiscreteIntegrator  SampleTime=Ts  SaturateOnIntegerOverflow=on  ICPrevOutput=DiscIntNeverNeededParam  ICPrevScaledInput=DiscIntNeverNeededParam
  Ld/Lq : Gain  Gain=Ld/Lq  SaturateOnIntegerOverflow=on
  Product1 : Product  SaturateOnIntegerOverflow=on  InputSameDT=on
  R/Lq : Gain  Gain=R/Lq  SaturateOnIntegerOverflow=on
  Sum1 : Sum  Inputs=---+  SaturateOnIntegerOverflow=on  InputSameDT=on
  lam/Lq : Gain  Gain=lam/Lq  SaturateOnIntegerOverflow=on
  iq : Outport  InitialOutput=0
  wires:
  Discrete-Time Integrator/1 -> iq/1, R/Lq/1
  we/1 -> lam/Lq/1, Product1/2
  vq/1 -> 1/Lq/1
  id/1 -> Product1/1
  1/Lq/1 -> Sum1/4
  Product1/1 -> Ld/Lq/1
  Sum1/1 -> Discrete-Time Integrator/1
  lam/Lq/1 -> Sum1/3
  Ld/Lq/1 -> Sum1/2
  R/Lq/1 -> Sum1/1

== system powerlib_modelsV2/Discrete/Three-Level Bridge/2-level GTO-IGBT Bridge  Logic (modified)/Diode Logic ==
  Vak : Inport  Port=1  LatchInput=off
  G : Inport  Port=2  LatchInput=off
  0 2 : Constant  Value=0
  1 : Logic
  Blocking Diodes : Subsystem
  Data Type  Conversion5 : DataTypeConversion  SaturateOnIntegerOverflow=on  RndMeth=Zero
  Logical Operator3 : Logic  Operator=NOT
  b6 : RelationalOperator  Operator=>  InputSameDT=on
  status : Outport  InitialOutput=0
  block : Outport  Port=2  InitialOutput=0
  wires:
  1/1 -> status/1
  Logical Operator3/1 -> 1/2
  Blocking Diodes/1(Block.D) -> block/1, Logical Operator3/1
  G/1 -> Blocking Diodes/1(G)
  0 2/1 -> b6/2
  Vak/1 -> b6/1
  b6/1 -> Data Type  Conversion5/1
  Data Type  Conversion5/1 -> 1/1

== system powerlib_modelsV2/Discrete/Three-Level Bridge/2-level GTO-IGBT Bridge  Logic (modified)/GTO Logic ==
  Vak : Inport  Port=1  LatchInput=off
  G : Inport  Port=2  LatchInput=off
  " " : RelationalOperator  Operator=>  InputSameDT=on
  "    " : Constant  Value=0
  ". " : Logic
  Data Type  Conversion1 : DataTypeConversion  SaturateOnIntegerOverflow=on  RndMeth=Zero
  Data Type  Conversion2 : DataTypeConversion  SaturateOnIntegerOverflow=on  RndMeth=Zero
  Data Type  Conversion3 : DataTypeConversion  SaturateOnIntegerOverflow=on  RndMeth=Zero
  Vpos : Constant  Value=0
  b : RelationalOperator  Operator=>  InputSameDT=on
  status : Outport  InitialOutput=0
  wires:
  ". "/1 -> status/1
  Vak/1 -> b/1
  Vpos/1 -> b/2
  G/1 -> " "/1
  b/1 -> Data Type  Conversion1/1
  Data Type  Conversion1/1 -> ". "/1
  " "/1 -> Data Type  Conversion2/1
  Data Type  Conversion2/1 -> ". "/2
  "    "/1 -> Data Type  Conversion3/1
  Data Type  Conversion3/1 -> " "/2

== system powerlib_modelsV2/Discrete/Three-Level Bridge/2-level GTO-IGBT Bridge  Logic (modified)/Vf  ==
  status_GTO : Inport  Port=1  LatchInput=off
  Switch : Switch  Threshold=0.5  SaturateOnIntegerOverflow=on  InputSameDT=on
  Vf device : Constant  Value=Vf*ones(nb_switch,1)
  Vf diode : Constant  Value=-Vfd*ones(nb_switch,1)
  Vf : Outport  InitialOutput=[0]
  wires:
  status_GTO/1 -> Switch/2
  Switch/1 -> Vf/1
  Vf diode/1 -> Switch/3
  Vf device/1 -> Switch/1

== system powerlib_modelsV2/Discrete/Three-Level Bridge/Sw3 (clamping diode) Logic/Note 3 ==
  G : Inport  Port=1  LatchInput=off
  Logical Operator : Logic  Operator=NOT
  Mux : Mux  Inputs=[nb_arm nb_arm]
  Pulse 1 step : Logic
  Select_BlockD : Selector  Elements=BlockDElements  InputPortWidth=nb_arm*2
  Unit Delay : UnitDelay  SampleTime=Ts
  Block.D : Outport
  wires:
  Unit Delay/1 -> Logical Operator/1
  Logical Operator/1 -> Pulse 1 step/1
  G/1 -> Unit Delay/1, Pulse 1 step/2
  Pulse 1 step/1 -> Mux/2, Mux/1  "Blocking"
  Mux/1 -> Select_BlockD/1
  Select_BlockD/1 -> Block.D/1

== system powerlib_modelsV2/Discrete/Three-Level Bridge/Sw3 (clamping diode) Logic/Note 4 ==
  pulses : Inport  Port=1  LatchInput=off
  D5_On : Inport  Port=2  LatchInput=off
  D6_On : Inport  Port=3  LatchInput=off
  Status_GTO : Inport  Port=4  LatchInput=off
  Demux : Demux  Outputs=[nb_arm nb_arm nb_arm nb_arm]
  Demux1 : Demux  Outputs=[nb_arm nb_arm]
  Logical Operator{,4,6,10} (4 alike) : Logic  Operator=NOT
  Logical Operator1 : Logic  Operator=NOR  Inputs=4
  Logical Operator{2..3,5,9} (4 alike) : Logic  Inputs=3
  Logical Operator7 : Logic  Operator=OR
  Logical Operator8 : Logic  Operator=OR
  Mux1 : Mux  Inputs=2
  Select_StatGTO : Selector  Elements=Trig12Elements  InputPortWidth=nb_arm*2
  Unit Delay{,1..3} (4 alike) : UnitDelay  SampleTime=Ts
  Trig12 : Outport
  wires:
  pulses/1 -> Demux/1
  D6_On/1 -> Unit Delay/1, Logical Operator/1
  Unit Delay/1 -> Logical Operator3/1
  Logical Operator/1 -> Logical Operator3/2
  D5_On/1 -> Logical Operator4/1, Unit Delay2/1
  Unit Delay2/1 -> Logical Operator5/2
  Logical Operator4/1 -> Logical Operator5/3
  Mux1/1 -> Trig12/1
  Demux/1 -> Logical Operator1/1
  Demux/2 -> Logical Operator1/2
  Demux/3 -> Logical Operator1/3
  Demux/4 -> Logical Operator1/4
  Logical Operator1/1 -> Logical Operator3/3, Logical Operator5/1, Logical Operator2/1, Logical Operator9/1
  Status_GTO/1 -> Select_StatGTO/1
  Logical Operator6/1 -> Logical Operator2/3
  Unit Delay1/1 -> Logical Operator2/2
  Logical Operator3/1 -> Logical Operator7/1
  Logical Operator7/1 -> Mux1/1
  Logical Operator5/1 -> Logical Operator8/1
  Logical Operator8/1 -> Mux1/2
  Select_StatGTO/1 -> Demux1/1
  Demux1/1 -> Unit Delay1/1, Logical Operator6/1
  Logical Operator10/1 -> Logical Operator9/3
  Demux1/2 -> Unit Delay3/1, Logical Operator10/1
  Unit Delay3/1 -> Logical Operator9/2
  Logical Operator2/1 -> Logical Operator8/2
  Logical Operator9/1 -> Logical Operator7/2

== system powerlib_modelsV2/Discrete/Three-Level Bridge/Sw3 (clamping diode) Logic/Vf Computation for Sw3 ==
  D5_On : Inport  Port=1  LatchInput=off
  Gain1 : Gain  Gain=-1  SaturateOnIntegerOverflow=on
  Gain2 : Gain  SaturateOnIntegerOverflow=on
  Switch : Switch  Threshold=0.5  SaturateOnIntegerOverflow=on  InputSameDT=on
  Vf device : Constant  Value=(Vf+Vfd)*ones(nb_arm,1)
  Vf : Outport
  wires:
  D5_On/1 -> Switch/2
  Gain2/1 -> Switch/3
  Gain1/1 -> Switch/1
  Vf device/1 -> Gain2/1, Gain1/1
  Switch/1 -> Vf/1
